simulink library "Lib_SUMOInterface"  (R2017b)
settings: Solver=ode45  StartTime=0.0  StopTime=10.0  RelTol=1e-3  EnableMultiTasking=on
settings Model: Creator=michaelstolz  LastModifiedBy=eldarkurtic
settings DataIOCC: LimitDataPoints=on  SaveFormat=StructureWithTime
settings OptimizationCC: LifeSpan=inf
settings DebuggingCC: FcnCallInpInsideContextMsg=warning  SFUnexpectedBacktrackingDiag=warning  SFNoUnconditionalDefaultTransitionDiag=warning  SFExecutionAtInitializationDiag=none
settings HardwareCC: ProdBitPerSizeT=32  ProdBitPerPtrDiffT=32  ProdWordSize=32  ProdHWDeviceType=Specified
settings ModelReferenceCC: PropagateSignalLabelsOutOfModel=off
settings CodeAppCC: StateflowObjectComments=on
settings GRTTargetCC: TargetLangStandard=C89/C90 (ANSI)
settings ConfigComp: CovMetricSettings=dw  CovHtmlReporting=on  CovSaveCumulativeToWorkspaceVar=on  CovSaveSingleToWorkspaceVar=on  CovExternalEMLEnable=off

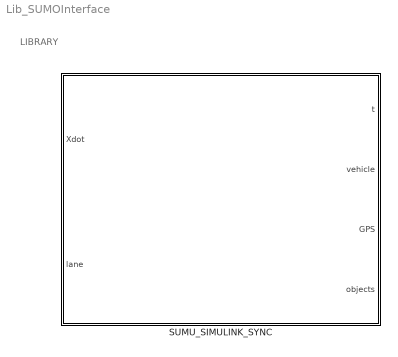
== system Lib_SUMOInterface ==
  note: LIBRARY
  SUMU_SIMULINK_SYNC : Subsystem  mask(SUMO Simulink Syncronisation){SumoTs_=0.02, EgoName_={'ego'}, SumoCfg_=data\tla_Example.sumocfg, SumoGui_=on, SumoIP_=127.0.0.1, SumoPort_=8873, SumoOptions_=, NumVehicles_=3, SensorRange_=0, NumTLights_=2}
      mask prompts: SumoTs_ "Sample time for SUMO in [s]"; EgoName_ "Ego vehicle name(s) in SUMO"; SumoCfg_ "SUMO config-file name. (delete for dialog)"; SumoGui_ "Select if the GUI is used or the command line executable."; SumoIP_ "Connection name (default '127.0.0.1')"; SumoPort_ "Port number for SUMO connection (deault 8873)."; SumoOptions_ "Additional command line options for sumo executable."; NumVehicles_ "Maximum number of traffic objects"; SensorRange_ "Detection range [m]. (values <=0 disables range checking)"; NumTLights_ "Maximum number of traffic lights"
      mask help:
      | This Block syncs a vehicle simulation in Simulink with a traffic simulation
      | in SUMO.
      |
      | Syncronisation is performed for one or more vehicle(s) called the
      | "ego"-vehicle(s).
      | The position and velocity information provided from vehicle simulation is
      | send to SUMO to move the corresponding vehicle in the traffic simulation
      | acordingly.
      |
      | Inputs:
      | X     [m] ...... horzintal position of vehicle to sync
      | Y     [m] ...... vertical position of vehicle to sync
      | dX/dt [m/s] .... horizontal velocity of vehicle to sync
      | dY/dt [m/s] .... horizontal velocity of vehicle to sync
      | T     [rad] .... orientation of vehicle to sync
      |                  ( OPTIONAL if sensors are used, otherwise set to NaN )
      | lane  [-] ...... lane of vehicle if in a multilane scenario
      |                  ( currently not used )
      | y_L   [m] ...... lateral offset of vehicle to sync
      |                  ( OPTIONAL if lane assignment shall be done, otherwise 0)
      |
      | Outputs:
      |  * t [s] ....... SUMO simulation time
      |                  (for checking and for traffic light trigger checks)
      |  * vehicle ..... information for ego vehicle(s) within a bus
      |  * GPS   ....... additional GPS information for ego vehicle(s) in a bus
      |  * objects ..... information regarding traffic objects in range in a bus
      |  * signals ..... information regarding traffic lights ahead in a bus
      |
      | Please read the help text for further information.
      mask Help:
      | MASK PARAMETERS:
      | 
      | The following mask parameters can be set, in order to control the behavior of the sync interface:
      | 
      | o) Ego vehicle names as strings in cell array. These names correspond to to the vehicle names in the SUMO config file which should be synced.
      | o) SUMO sample time in [s]: this is the fixed time step SUMO is updated
      | o) SUMO interface IP adress and port number
      | o) SUMO graphical mode activation/diactivation: set wheter to use the gui or command line tool only
      | o) SUMO configuartion file name: better use relative paths for interoperability
      | o) SUMO additional command line parameters: add options to e.g. log something
      | 
      | o) Maximum number of traffic objects to be send at output
      | o) Maximum range around vehicle for traffic objects to be relevant
      | 
      | o) Maximum number of traffic lights to be send at output
      | 
      | POSITION SYNCRONISATION:
      | 
      | Due to several shortcomings of the used TraCi-Interface from SUMO direct position synchronization could not be used in general, therefore
      | indirect synchronization via velocity is used.
      | 
      | Velocity information is used as main syncronization method. Position info is used additionally to correct velocity to improve matching and avoid
      | drifting.
      | Note that setting velocity of the ego-vehicle for synchronization will not in all cases take imidiate effect due to acceleration limits and driver
      | model limitations. However a lot of measures have been taken in order to set the velocity directly:
      |   * min/max acceleration rates have been set to +-1000
      |   * time const of driver model has been set to 0
      |   * speed mode has been set to 0 --> ignoring a lot of speedlimits
      |   * --ignore-accidents has been used in command line
      | 
      | 
      | 
      | INTERFACES:
      | 
      | t : scalar time of SUMO-simulation in seconds.
      | 
      | vehicle : a bus holding ego vehicles informations
      |     * X position [m]
      |     * Y position [m]
      |     * V velocity [m/s]
      |     * T angle [rad] (anticlockwise starting from x)
      |     * D traveled distance [m]
      | 
      | GPS: a bus holding information from FIRST ego car and its road segment
      | 
      | objects: a bus holding information from traffic objects in the given range (mask parameter) of the FIRST ego car. Note the bus signals stay the same, the dimension of each signal will depend on the selected maximum number of traffic objects (mask parameter)
      |  flag_objects : 0=off, 1=on, 2=on and new
      | distx_objects : the distance of the object measured in coordinate system of the FIRST ego vehicle along the x axis
      | disty_objects : the distance of the object measured in coordinate system of the FIRST ego vehicle along the y axis
      | velx_objects : the velocity (absolute!) of the object measured in coordinate system of the FIRST ego vehicle along the x axis
      | vely_objects : the velocity (absolute!) of the object measured in coordinate system of the FIRST ego vehicle along the y axis
      | signal_objects : the signal state of the traffic object. see SUMO documentation for details (brake signal, lane change signal, ...)
      | 
      | signals: a bus holding information from traffic lights ahead of the FIRST ego vehicle. Note the bus signals stay the same, the dimension of each signal will depend on the selected maximum number of traffic lights (mask parameter).
      | flag_signals     : 0=off, 1=on
      | distance_signals : driving distance along the road to the traffic light
      | tswitch_signals  : (absolute) time instance of next switching in seconds
      | phase_signals    : current phase (0 for green, 1 for red)
      | red_signals      : duration of red phase in seconds
      | green_signals    : duration of green phase in seconds
      mask TypeOptions SumoTs_: SIM_SYNC/SumoTs
      mask TypeOptions EgoName_: SIM_SYNC/EgoName
      mask Callback EgoName_:
      | if isempty(get_param(gcb,'EgoName_')),
      |     set_param(gcb, 'EgoName_','{''ego''}');
      | end
      mask TypeOptions SumoCfg_: SIM_SYNC/SumoCfg
      mask Callback SumoCfg_:
      | if isempty(get_param(gcb,'SumoCfg_')),
      |     [myvars.fileName, myvars.filePath] = uigetfile('*.sumocfg','Select a SUMO config File');
      |     if ~isequal(myvars.fileName,0),
      |         set_param(gcb, 'SumoCfg_',fullfile(myvars.filePath,myvars.fileName));
      |     end
      |     clear myvars
      | end
      mask TypeOptions SumoGui_: SIM_SYNC/SumoGui
      mask TypeOptions SumoIP_: SIM_SYNC/SumoIP
      mask Callback SumoIP_:
      | if isempty(get_param(gcb,'SumoIP_')),
      |     set_param(gcb, 'SumoIP_','127.0.0.1');
      | end
      mask TypeOptions SumoPort_: SIM_SYNC/SumoPort
      mask Callback SumoPort_:
      | if isempty(get_param(gcb,'SumoPort_')),
      |     set_param(gcb, 'SumoPort_','8873');
      | end
      mask TypeOptions SumoOptions_: SIM_SYNC/SumoOptions
      mask TypeOptions NumVehicles_: SIM_SYNC/NumVehicles
      mask Callback NumVehicles_:
      | if isempty(get_param(gcb,'NumVehicles_')),
      |     set_param(gcb, 'NumVehicles_','0');
      | end
      mask TypeOptions SensorRange_: SIM_SYNC/SensorRange
      mask TypeOptions NumTLights_: SIM_SYNC/NumTLights
      mask Callback NumTLights_:
      | if isempty(get_param(gcb,'NumTLights_')),
      |     set_param(gcb, 'NumTLights_','0');
      | end
      mask DialogControl ParameterTabVar0 Prompt: SIMULATION
      mask DialogControl ParameterTabVar01 Prompt: SUMO
      mask DialogControl ParameterTabVar012 Prompt: OBJECTS
      mask DialogControl ParameterTabVar0123 Prompt: SIGNALS
      mask Display:
      | text(.5,.8,'\fontname{palatino}\fontsize{15}\bf Simulink-SUMO SYNC',...
      |       'HorizontalAlignment','center','texmode','on');
      | text(.5,.6,['sample rate = ',sprintf('%4.2f [s]',SumoTs_)],...
      |       'HorizontalAlignment','center','texmode','on');
      | text(.5,.4,['ego vehicle name : ',sprintf('"%s" ',EgoName_{:})],...
      |       'HorizontalAlignment','center','texmode','off');
      | text(.5,.2,sprintf('"%s"',SumoCfg_),...
      |       'HorizontalAlignment','center','texmode','off');
      | port_label('input',1,'vel [m/s]');
      | 
      | port_label('input',2,'lane  [-]');
      | 
      | 
      | port_label('output',1,'t');
      | port_label('output',2,'vehicle');
      | port_label('output',3,'GPS');
      | port_label('output',4,sprintf('%d objects',NumVehicles_));

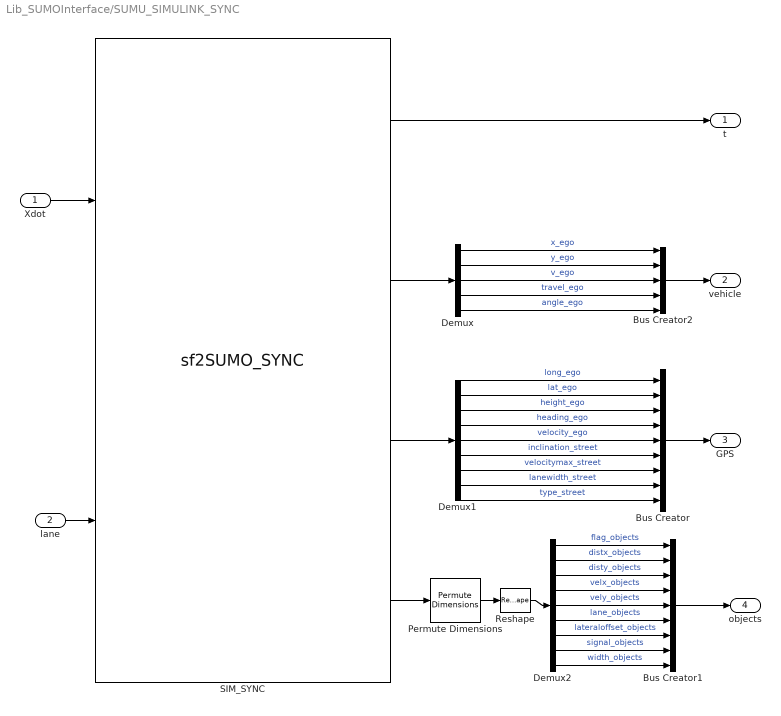
== system Lib_SUMOInterface/SUMU_SIMULINK_SYNC ==
  Xdot : Inport
  lane : Inport  Port=2
  Bus Creator : BusCreator  Inputs=9
  Bus Creator1 : BusCreator  Inputs=9
  Bus Creator2 : BusCreator  Inputs=5
  Demux : Demux  Outputs=5
  Demux1 : Demux  Outputs=9
  Demux2 : Demux  Outputs=[-1,-1,-1,-1,-1,-1,-1,-1,-1]
  Permute Dimensions : PermuteDimensions
  Reshape : Reshape
  SIM_SYNC : M-S-Function  FunctionName=sf2SUMO_SYNC  Parameters=SumoTs,EgoName,NumVehicles,SumoCfg,SumoIP,SumoPort,SumoGui,SumoOptions,NumTLights,SensorRange  mask(SUMO Simulink Syncronisation){SumoTs=SumoTs_, EgoName=EgoName_, SumoPort=SumoPort_, SumoIP=127.0.0.1, SumoCfg=data\tla_Example.sumocfg, SumoGui=on, SumoOptions=, NumVehicles=NumVehicles_, SensorRange=SensorRange_, NumTLights=NumTLights_}
      mask prompts: SumoTs "Sample time for SUMO in [s]"; EgoName "Ego vehicle name(s) in SUMO ( default {'ego'} )"; SumoPort "Port number for SUMO connection (default 8873)"; SumoIP "Connection name (default: '127.0.0.1')"; SumoCfg "Full SUMO config-file name"; SumoGui "Select if the GUI is used or the command line tool."; SumoOptions "Additional command line options for SUMO:"; NumVehicles "Maximum number of traffic objects."; SensorRange "Detection range [m]"; NumTLights "Maximum number of traffic lights"
      mask Callback EgoName:
      | if isempty(get_param(gcb,'EgoName')),
      |     set_param(gcb, 'EgoName','{''ego''}');
      | end
      mask Callback SumoPort:
      | if isempty(get_param(gcb,'SumoPort')),
      |     set_param(gcb, 'SumoPort','8873');
      | end
      mask Callback SumoIP:
      | if isempty(get_param(gcb,'SumoIP')),
      |     set_param(gcb, 'SumoIP','127.0.0.1');
      | end
      mask Callback SumoCfg:
      | if isempty(get_param(gcb,'SumoCfg')),
      |     [myvars.fileName, myvars.filePath] = uigetfile('*.sumocfg','Select a SUMO config File');
      |     if ~isequal(myvars.fileName,0),
      |         set_param(gcb, 'SumoCfg',fullfile(myvars.filePath,myvars.fileName));
      |     end
      |     clear myvars
      | end
      mask DialogControl ParameterTabVar0 Prompt: SIMULATION
      mask DialogControl ParameterTabVar01 Prompt: SUMO
      mask DialogControl ParameterTabVar012 Prompt: SENSORS
      mask DialogControl ParameterTabVar0123 Prompt: TRAFFIC LIGHTS
      mask Display:
      | text(.5,.8,'\fontname{palatino}\fontsize{15}\bf Simulink-SUMO SYNC',...
      |       'HorizontalAlignment','center','texmode','on');
      | text(.5,.6,['sample rate = ',sprintf('%4.2f [s]',SumoTs)],...
      |       'HorizontalAlignment','center','texmode','on');
      | text(.5,.4,['ego vehicle name : ',sprintf('"%s" ',EgoName{:})],...
      |       'HorizontalAlignment','center','texmode','off');
      | text(.5,.2,sprintf('"%s"',SumoCfg),...
      |       'HorizontalAlignment','center','texmode','off');
      | 
      | port_label('input',1,'ds/dt [m/s]');
      | 
      | port_label('input',2,'lane  [-]');
      | 
      | 
      | port_label('output',1,'t');
      | port_label('output',2,'vehicle');
      | port_label('output',3,'GPS');
      | port_label('output',4,sprintf('%d objects',NumVehicles));
  t : Outport
  vehicle : Outport  Port=2
  GPS : Outport  Port=3
  objects : Outport  Port=4
  wires:
  Bus Creator1/1 -> objects/1
  lane/1 -> SIM_SYNC/2
  Bus Creator/1 -> GPS/1
  Bus Creator2/1 -> vehicle/1
  Xdot/1 -> SIM_SYNC/1
  SIM_SYNC/1 -> t/1
  Demux/5 -> Bus Creator2/5  "angle_ego"
  Demux/4 -> Bus Creator2/4  "travel_ego"
  Permute Dimensions/1 -> Reshape/1
  Reshape/1 -> Demux2/1
  Demux2/8 -> Bus Creator1/8  "signal_objects"
  Demux2/7 -> Bus Creator1/7  "lateraloffset_objects"
  Demux2/6 -> Bus Creator1/6  "lane_objects"
  Demux2/5 -> Bus Creator1/5  "vely_objects"
  Demux2/4 -> Bus Creator1/4  "velx_objects"
  Demux2/3 -> Bus Creator1/3  "disty_objects"
  Demux2/2 -> Bus Creator1/2  "distx_objects"
  Demux2/1 -> Bus Creator1/1  "flag_objects"
  Demux1/9 -> Bus Creator/9  "type_street"
  Demux1/8 -> Bus Creator/8  "lanewidth_street"
  Demux1/7 -> Bus Creator/7  "velocitymax_street"
  Demux1/6 -> Bus Creator/6  "inclination_street"
  Demux1/5 -> Bus Creator/5  "velocity_ego"
  Demux1/4 -> Bus Creator/4  "heading_ego"
  Demux1/3 -> Bus Creator/3  "height_ego"
  Demux1/2 -> Bus Creator/2  "lat_ego"
  Demux1/1 -> Bus Creator/1  "long_ego"
  SIM_SYNC/4 -> Permute Dimensions/1
  SIM_SYNC/3 -> Demux1/1
  Demux/3 -> Bus Creator2/3  "v_ego"
  Demux/1 -> Bus Creator2/1  "x_ego"
  Demux/2 -> Bus Creator2/2  "y_ego"
  SIM_SYNC/2 -> Demux/1
  Demux2/9 -> Bus Creator1/9  "width_objects"
